simulink model "gm_Model"  (R2025a)
settings: Solver=FixedStepDiscrete  StartTime=0.0  StopTime=80000/fs_in  RelTol=1e-3
undefined symbols (not defined in the file or in its folder): a, b, b_fixp, beta_retanh, c, cos_omega, cos_omega_fixp, diag_count, exp_omega, exp_omega_fixp, fixp_chebacc_frac, fixp_chebacc_ws, fixp_dsp_ws, fixp_eig_frac, fixp_eig_ws, fs_in, group_size, hann_table_fixp, image_seed, image_seed_fixp, J_ROM, k, K_ROM, lap_diags, lap_main, lap_main_fi, lap_offsets, lap_offsets_fi, lap_rest, lap_rest_fi, laplacian_diags_main, laplacian_diags_offsets, laplacian_diags_rest, lut_norm_x, lut_norm_y, magnitude, n_ch, n_layer, n_px, n_px_fi, nf, norm_gain_floor, power_iters, power_norm_scaling_factor_fixp, tau, tau_fixp, theta, theta_fixp
libraries: simulink x59, hdlsllib x36, hdlstreaminglib x4, hdlmdlgenlib x1, matrix_library x1, dspvision x1
(part 7 of 8)

== system gm_Model/DUT_Test/Goertzel/EnabledGoertzel/crp_temp_streamed2/Serializer_Subnetwork1 ==
  in0 : Inport  OutDataTypeStr=fixdt(1, 18, 13)  PortDimensions=[1 48]  SampleTime=3.125e-07
  in1 : Inport  Port=2  OutDataTypeStr=fixdt(0, 6, 0)  SampleTime=3.125e-07
  ratechange_splitcomp : Demux  Outputs=48
  splitcomp_multiport : MultiPortSwitch  DataPortOrder=Zero-based contiguous  Inputs=48  DiagnosticForDefault=None  zeroidx=on  OutDataTypeStr=fixdt(1, 18, 13)  SampleTime=3.125e-07  SaturateOnIntegerOverflow=off  InputSameDT=off
  out0 : Outport  OutDataTypeStr=fixdt(1, 18, 13)  SampleTime=3.125e-07
  wires:
  in0/1 -> ratechange_splitcomp/1
  in1/1 -> splitcomp_multiport/1
  ratechange_splitcomp/1 -> splitcomp_multiport/2
  ratechange_splitcomp/2 -> splitcomp_multiport/3
  ratechange_splitcomp/3 -> splitcomp_multiport/4
  ratechange_splitcomp/4 -> splitcomp_multiport/5
  ratechange_splitcomp/8 -> splitcomp_multiport/9
  ratechange_splitcomp/7 -> splitcomp_multiport/8
  ratechange_splitcomp/5 -> splitcomp_multiport/6
  ratechange_splitcomp/6 -> splitcomp_multiport/7
  ratechange_splitcomp/12 -> splitcomp_multiport/13
  ratechange_splitcomp/11 -> splitcomp_multiport/12
  ratechange_splitcomp/10 -> splitcomp_multiport/11
  ratechange_splitcomp/9 -> splitcomp_multiport/10
  ratechange_splitcomp/16 -> splitcomp_multiport/17
  ratechange_splitcomp/15 -> splitcomp_multiport/16
  ratechange_splitcomp/14 -> splitcomp_multiport/15
  ratechange_splitcomp/13 -> splitcomp_multiport/14
  splitcomp_multiport/1 -> out0/1
  ratechange_splitcomp/20 -> splitcomp_multiport/21
  ratechange_splitcomp/19 -> splitcomp_multiport/20
  ratechange_splitcomp/18 -> splitcomp_multiport/19
  ratechange_splitcomp/17 -> splitcomp_multiport/18
  ratechange_splitcomp/45 -> splitcomp_multiport/46
  ratechange_splitcomp/44 -> splitcomp_multiport/45
  ratechange_splitcomp/43 -> splitcomp_multiport/44
  ratechange_splitcomp/42 -> splitcomp_multiport/43
  ratechange_splitcomp/24 -> splitcomp_multiport/25
  ratechange_splitcomp/23 -> splitcomp_multiport/24
  ratechange_splitcomp/22 -> splitcomp_multiport/23
  ratechange_splitcomp/21 -> splitcomp_multiport/22
  ratechange_splitcomp/48 -> splitcomp_multiport/49
  ratechange_splitcomp/47 -> splitcomp_multiport/48
  ratechange_splitcomp/46 -> splitcomp_multiport/47
  ratechange_splitcomp/28 -> splitcomp_multiport/29
  ratechange_splitcomp/27 -> splitcomp_multiport/28
  ratechange_splitcomp/26 -> splitcomp_multiport/27
  ratechange_splitcomp/25 -> splitcomp_multiport/26
  ratechange_splitcomp/32 -> splitcomp_multiport/33
  ratechange_splitcomp/31 -> splitcomp_multiport/32
  ratechange_splitcomp/30 -> splitcomp_multiport/31
  ratechange_splitcomp/29 -> splitcomp_multiport/30
  ratechange_splitcomp/36 -> splitcomp_multiport/37
  ratechange_splitcomp/35 -> splitcomp_multiport/36
  ratechange_splitcomp/34 -> splitcomp_multiport/35
  ratechange_splitcomp/33 -> splitcomp_multiport/34
  ratechange_splitcomp/39 -> splitcomp_multiport/40
  ratechange_splitcomp/38 -> splitcomp_multiport/39
  ratechange_splitcomp/37 -> splitcomp_multiport/38
  ratechange_splitcomp/40 -> splitcomp_multiport/41
  ratechange_splitcomp/41 -> splitcomp_multiport/42

== system gm_Model/DUT_Test/Goertzel/EnabledGoertzel/crp_temp_streamed2/Switch_out1_bypass ==
  in0 : Inport  OutDataTypeStr=fixdt(1, 18, 13)  SampleTime=3.125e-07
  in1 : Inport  Port=2  OutDataTypeStr=boolean  SampleTime=3.125e-07
  Switch_out1_enb : Switch  Criteria=u2 ~= 0  Threshold=double(0)  OutDataTypeStr=fixdt(1, 18, 13)  SampleTime=3.125e-07  SaturateOnIntegerOverflow=off  InputSameDT=off
  Switch_out1_state : Delay  DelayLength=double(1)  InitialCondition=0  SampleTime=3.125e-07
  out0 : Outport  OutDataTypeStr=fixdt(1, 18, 13)  SampleTime=3.125e-07
  wires:
  in1/1 -> Switch_out1_enb/2
  in0/1 -> Switch_out1_enb/1
  Switch_out1_state/1 -> Switch_out1_enb/3
  Switch_out1_enb/1 -> Switch_out1_state/1, out0/1

== system gm_Model/DUT_Test/Goertzel/EnabledGoertzel/crp_temp_streamed2/counter ==
  globalSchedule : EnablePort  OutDataTypeStr=boolean
  ctr_0_47 : hdlsllib/Sources/HDL Counter  CountType=Count limited  CountInit=double(0)  CountStep=double(1)  CountMax=double(47)  CountFromType=Initial value  CountFrom=double(0)  CountResetPort=off  CountLoadPort=off  CountEnbPort=off  CountDirPort=off  CountHitOutputPort=off  CountDataType=Unsigned  CountWordLen=6  CountFracLen=0  CountSampTime=3.125e-07
  out0 : Outport  OutDataTypeStr=fixdt(0, 6, 0)  SampleTime=3.125e-07  InitialOutput=0
  wires:
  ctr_0_47/1 -> out0/1

== system gm_Model/DUT_Test/Goertzel/EnabledGoertzel/crp_temp_streamed2/tappedDelay ==
  in0 : Inport  OutDataTypeStr=fixdt(1, 18, 13)  SampleTime=3.125e-07
  globalSchedule : EnablePort  OutDataTypeStr=boolean
  StateControl : StateControl  StateControl=Synchronous
  tapped_delay : simulink/Discrete/Tapped Delay  vinit=0  samptime=-1  NumDelays=double(47)  DelayOrder=Oldest  includeCurrent=off
  out0 : Outport  OutDataTypeStr=fixdt(1, 18, 13)  PortDimensions=[47]  SampleTime=3.125e-07  InitialOutput=0
  wires:
  in0/1 -> tapped_delay/1
  tapped_delay/1 -> out0/1

== system gm_Model/DUT_Test/Goertzel/EnabledGoertzel/streaming_partition_streamed/Serializer_Subnetwork ==
  in0 : Inport  OutDataTypeStr=fixdt(1, 18, 13)  PortDimensions=[1 48]  SampleTime=3.125e-07
  in1 : Inport  Port=2  OutDataTypeStr=fixdt(0, 6, 0)  SampleTime=3.125e-07
  ratechange_splitcomp : Demux  Outputs=48
  splitcomp_multiport : MultiPortSwitch  DataPortOrder=Zero-based contiguous  Inputs=48  DiagnosticForDefault=None  zeroidx=on  OutDataTypeStr=fixdt(1, 18, 13)  SampleTime=3.125e-07  SaturateOnIntegerOverflow=off  InputSameDT=off
  out0 : Outport  OutDataTypeStr=fixdt(1, 18, 13)  SampleTime=3.125e-07
  wires:
  in0/1 -> ratechange_splitcomp/1
  in1/1 -> splitcomp_multiport/1
  ratechange_splitcomp/1 -> splitcomp_multiport/2
  ratechange_splitcomp/2 -> splitcomp_multiport/3
  ratechange_splitcomp/3 -> splitcomp_multiport/4
  ratechange_splitcomp/7 -> splitcomp_multiport/8
  ratechange_splitcomp/4 -> splitcomp_multiport/5
  ratechange_splitcomp/5 -> splitcomp_multiport/6
  ratechange_splitcomp/6 -> splitcomp_multiport/7
  ratechange_splitcomp/11 -> splitcomp_multiport/12
  ratechange_splitcomp/10 -> splitcomp_multiport/11
  ratechange_splitcomp/9 -> splitcomp_multiport/10
  ratechange_splitcomp/8 -> splitcomp_multiport/9
  ratechange_splitcomp/15 -> splitcomp_multiport/16
  ratechange_splitcomp/14 -> splitcomp_multiport/15
  ratechange_splitcomp/13 -> splitcomp_multiport/14
  ratechange_splitcomp/12 -> splitcomp_multiport/13
  ratechange_splitcomp/19 -> splitcomp_multiport/20
  ratechange_splitcomp/18 -> splitcomp_multiport/19
  ratechange_splitcomp/17 -> splitcomp_multiport/18
  ratechange_splitcomp/16 -> splitcomp_multiport/17
  ratechange_splitcomp/23 -> splitcomp_multiport/24
  ratechange_splitcomp/22 -> splitcomp_multiport/23
  ratechange_splitcomp/21 -> splitcomp_multiport/22
  ratechange_splitcomp/20 -> splitcomp_multiport/21
  ratechange_splitcomp/27 -> splitcomp_multiport/28
  ratechange_splitcomp/26 -> splitcomp_multiport/27
  ratechange_splitcomp/25 -> splitcomp_multiport/26
  ratechange_splitcomp/24 -> splitcomp_multiport/25
  ratechange_splitcomp/31 -> splitcomp_multiport/32
  ratechange_splitcomp/30 -> splitcomp_multiport/31
  ratechange_splitcomp/29 -> splitcomp_multiport/30
  ratechange_splitcomp/28 -> splitcomp_multiport/29
  ratechange_splitcomp/35 -> splitcomp_multiport/36
  ratechange_splitcomp/34 -> splitcomp_multiport/35
  ratechange_splitcomp/33 -> splitcomp_multiport/34
  ratechange_splitcomp/32 -> splitcomp_multiport/33
  ratechange_splitcomp/39 -> splitcomp_multiport/40
  ratechange_splitcomp/38 -> splitcomp_multiport/39
  ratechange_splitcomp/37 -> splitcomp_multiport/38
  ratechange_splitcomp/36 -> splitcomp_multiport/37
  ratechange_splitcomp/43 -> splitcomp_multiport/44
  ratechange_splitcomp/42 -> splitcomp_multiport/43
  ratechange_splitcomp/41 -> splitcomp_multiport/42
  ratechange_splitcomp/40 -> splitcomp_multiport/41
  ratechange_splitcomp/47 -> splitcomp_multiport/48
  ratechange_splitcomp/46 -> splitcomp_multiport/47
  ratechange_splitcomp/45 -> splitcomp_multiport/46
  ratechange_splitcomp/44 -> splitcomp_multiport/45
  ratechange_splitcomp/48 -> splitcomp_multiport/49
  splitcomp_multiport/1 -> out0/1

== system gm_Model/DUT_Test/Goertzel/EnabledGoertzel/streaming_partition_streamed/Serializer_Subnetwork1 ==
  in0 : Inport  OutDataTypeStr=fixdt(1, 18, 13)  PortDimensions=[1 48]  SampleTime=3.125e-07
  in1 : Inport  Port=2  OutDataTypeStr=fixdt(0, 6, 0)  SampleTime=3.125e-07
  ratechange_splitcomp : Demux  Outputs=48
  splitcomp_multiport : MultiPortSwitch  DataPortOrder=Zero-based contiguous  Inputs=48  DiagnosticForDefault=None  zeroidx=on  OutDataTypeStr=fixdt(1, 18, 13)  SampleTime=3.125e-07  SaturateOnIntegerOverflow=off  InputSameDT=off
  out0 : Outport  OutDataTypeStr=fixdt(1, 18, 13)  SampleTime=3.125e-07
  wires:
  in0/1 -> ratechange_splitcomp/1
  in1/1 -> splitcomp_multiport/1
  ratechange_splitcomp/1 -> splitcomp_multiport/2
  ratechange_splitcomp/2 -> splitcomp_multiport/3
  ratechange_splitcomp/3 -> splitcomp_multiport/4
  ratechange_splitcomp/4 -> splitcomp_multiport/5
  ratechange_splitcomp/8 -> splitcomp_multiport/9
  ratechange_splitcomp/7 -> splitcomp_multiport/8
  ratechange_splitcomp/5 -> splitcomp_multiport/6
  ratechange_splitcomp/6 -> splitcomp_multiport/7
  ratechange_splitcomp/12 -> splitcomp_multiport/13
  ratechange_splitcomp/11 -> splitcomp_multiport/12
  ratechange_splitcomp/10 -> splitcomp_multiport/11
  ratechange_splitcomp/9 -> splitcomp_multiport/10
  ratechange_splitcomp/16 -> splitcomp_multiport/17
  ratechange_splitcomp/15 -> splitcomp_multiport/16
  ratechange_splitcomp/14 -> splitcomp_multiport/15
  ratechange_splitcomp/13 -> splitcomp_multiport/14
  ratechange_splitcomp/20 -> splitcomp_multiport/21
  ratechange_splitcomp/19 -> splitcomp_multiport/20
  ratechange_splitcomp/18 -> splitcomp_multiport/19
  ratechange_splitcomp/17 -> splitcomp_multiport/18
  ratechange_splitcomp/24 -> splitcomp_multiport/25
  ratechange_splitcomp/23 -> splitcomp_multiport/24
  ratechange_splitcomp/22 -> splitcomp_multiport/23
  ratechange_splitcomp/21 -> splitcomp_multiport/22
  ratechange_splitcomp/28 -> splitcomp_multiport/29
  ratechange_splitcomp/27 -> splitcomp_multiport/28
  ratechange_splitcomp/26 -> splitcomp_multiport/27
  ratechange_splitcomp/25 -> splitcomp_multiport/26
  ratechange_splitcomp/32 -> splitcomp_multiport/33
  ratechange_splitcomp/31 -> splitcomp_multiport/32
  ratechange_splitcomp/30 -> splitcomp_multiport/31
  ratechange_splitcomp/29 -> splitcomp_multiport/30
  ratechange_splitcomp/36 -> splitcomp_multiport/37
  ratechange_splitcomp/35 -> splitcomp_multiport/36
  ratechange_splitcomp/34 -> splitcomp_multiport/35
  ratechange_splitcomp/33 -> splitcomp_multiport/34
  ratechange_splitcomp/39 -> splitcomp_multiport/40
  ratechange_splitcomp/38 -> splitcomp_multiport/39
  ratechange_splitcomp/37 -> splitcomp_multiport/38
  ratechange_splitcomp/40 -> splitcomp_multiport/41
  ratechange_splitcomp/41 -> splitcomp_multiport/42
  ratechange_splitcomp/45 -> splitcomp_multiport/46
  ratechange_splitcomp/44 -> splitcomp_multiport/45
  ratechange_splitcomp/43 -> splitcomp_multiport/44
  ratechange_splitcomp/42 -> splitcomp_multiport/43
  ratechange_splitcomp/48 -> splitcomp_multiport/49
  ratechange_splitcomp/47 -> splitcomp_multiport/48
  ratechange_splitcomp/46 -> splitcomp_multiport/47
  splitcomp_multiport/1 -> out0/1

== system gm_Model/DUT_Test/Goertzel/EnabledGoertzel/streaming_partition_streamed/Serializer_Subnetwork2 ==
  in0 : Inport  OutDataTypeStr=fixdt(1, 12, 11)  PortDimensions=[1 48]  SampleTime=3.125e-07
  in1 : Inport  Port=2  OutDataTypeStr=fixdt(0, 6, 0)  SampleTime=3.125e-07
  ratechange_splitcomp : Demux  Outputs=48
  splitcomp_multiport : MultiPortSwitch  DataPortOrder=Zero-based contiguous  Inputs=48  DiagnosticForDefault=None  zeroidx=on  OutDataTypeStr=fixdt(1, 12, 11)  SampleTime=3.125e-07  SaturateOnIntegerOverflow=off  InputSameDT=off
  out0 : Outport  OutDataTypeStr=fixdt(1, 12, 11)  SampleTime=3.125e-07
  wires:
  ratechange_splitcomp/47 -> splitcomp_multiport/48
  ratechange_splitcomp/46 -> splitcomp_multiport/47
  ratechange_splitcomp/45 -> splitcomp_multiport/46
  ratechange_splitcomp/44 -> splitcomp_multiport/45
  in0/1 -> ratechange_splitcomp/1
  in1/1 -> splitcomp_multiport/1
  ratechange_splitcomp/1 -> splitcomp_multiport/2
  ratechange_splitcomp/2 -> splitcomp_multiport/3
  ratechange_splitcomp/43 -> splitcomp_multiport/44
  ratechange_splitcomp/42 -> splitcomp_multiport/43
  ratechange_splitcomp/3 -> splitcomp_multiport/4
  ratechange_splitcomp/4 -> splitcomp_multiport/5
  ratechange_splitcomp/5 -> splitcomp_multiport/6
  ratechange_splitcomp/6 -> splitcomp_multiport/7
  ratechange_splitcomp/10 -> splitcomp_multiport/11
  ratechange_splitcomp/9 -> splitcomp_multiport/10
  ratechange_splitcomp/8 -> splitcomp_multiport/9
  ratechange_splitcomp/7 -> splitcomp_multiport/8
  ratechange_splitcomp/14 -> splitcomp_multiport/15
  ratechange_splitcomp/13 -> splitcomp_multiport/14
  ratechange_splitcomp/12 -> splitcomp_multiport/13
  ratechange_splitcomp/11 -> splitcomp_multiport/12
  splitcomp_multiport/1 -> out0/1
  ratechange_splitcomp/18 -> splitcomp_multiport/19
  ratechange_splitcomp/17 -> splitcomp_multiport/18
  ratechange_splitcomp/16 -> splitcomp_multiport/17
  ratechange_splitcomp/15 -> splitcomp_multiport/16
  ratechange_splitcomp/22 -> splitcomp_multiport/23
  ratechange_splitcomp/21 -> splitcomp_multiport/22
  ratechange_splitcomp/20 -> splitcomp_multiport/21
  ratechange_splitcomp/19 -> splitcomp_multiport/20
  ratechange_splitcomp/26 -> splitcomp_multiport/27
  ratechange_splitcomp/25 -> splitcomp_multiport/26
  ratechange_splitcomp/24 -> splitcomp_multiport/25
  ratechange_splitcomp/23 -> splitcomp_multiport/24
  ratechange_splitcomp/30 -> splitcomp_multiport/31
  ratechange_splitcomp/29 -> splitcomp_multiport/30
  ratechange_splitcomp/28 -> splitcomp_multiport/29
  ratechange_splitcomp/27 -> splitcomp_multiport/28
  ratechange_splitcomp/34 -> splitcomp_multiport/35
  ratechange_splitcomp/33 -> splitcomp_multiport/34
  ratechange_splitcomp/32 -> splitcomp_multiport/33
  ratechange_splitcomp/31 -> splitcomp_multiport/32
  ratechange_splitcomp/38 -> splitcomp_multiport/39
  ratechange_splitcomp/37 -> splitcomp_multiport/38
  ratechange_splitcomp/36 -> splitcomp_multiport/37
  ratechange_splitcomp/35 -> splitcomp_multiport/36
  ratechange_splitcomp/39 -> splitcomp_multiport/40
  ratechange_splitcomp/40 -> splitcomp_multiport/41
  ratechange_splitcomp/41 -> splitcomp_multiport/42
  ratechange_splitcomp/48 -> splitcomp_multiport/49

== system gm_Model/DUT_Test/Goertzel/EnabledGoertzel/streaming_partition_streamed/Serializer_Subnetwork3 ==
  in0 : Inport  OutDataTypeStr=fixdt(1, 18, 13)  PortDimensions=[1 48]  SampleTime=3.125e-07
  in1 : Inport  Port=2  OutDataTypeStr=fixdt(0, 6, 0)  SampleTime=3.125e-07
  ratechange_splitcomp : Demux  Outputs=48
  splitcomp_multiport : MultiPortSwitch  DataPortOrder=Zero-based contiguous  Inputs=48  DiagnosticForDefault=None  zeroidx=on  OutDataTypeStr=fixdt(1, 18, 13)  SampleTime=3.125e-07  SaturateOnIntegerOverflow=off  InputSameDT=off
  out0 : Outport  OutDataTypeStr=fixdt(1, 18, 13)  SampleTime=3.125e-07
  wires:
  in0/1 -> ratechange_splitcomp/1
  in1/1 -> splitcomp_multiport/1
  ratechange_splitcomp/1 -> splitcomp_multiport/2
  ratechange_splitcomp/2 -> splitcomp_multiport/3
  ratechange_splitcomp/3 -> splitcomp_multiport/4
  ratechange_splitcomp/4 -> splitcomp_multiport/5
  ratechange_splitcomp/8 -> splitcomp_multiport/9
  ratechange_splitcomp/7 -> splitcomp_multiport/8
  ratechange_splitcomp/5 -> splitcomp_multiport/6
  ratechange_splitcomp/6 -> splitcomp_multiport/7
  ratechange_splitcomp/12 -> splitcomp_multiport/13
  ratechange_splitcomp/11 -> splitcomp_multiport/12
  ratechange_splitcomp/10 -> splitcomp_multiport/11
  ratechange_splitcomp/9 -> splitcomp_multiport/10
  ratechange_splitcomp/16 -> splitcomp_multiport/17
  ratechange_splitcomp/15 -> splitcomp_multiport/16
  ratechange_splitcomp/14 -> splitcomp_multiport/15
  ratechange_splitcomp/13 -> splitcomp_multiport/14
  ratechange_splitcomp/20 -> splitcomp_multiport/21
  ratechange_splitcomp/19 -> splitcomp_multiport/20
  ratechange_splitcomp/18 -> splitcomp_multiport/19
  ratechange_splitcomp/17 -> splitcomp_multiport/18
  ratechange_splitcomp/24 -> splitcomp_multiport/25
  ratechange_splitcomp/23 -> splitcomp_multiport/24
  ratechange_splitcomp/22 -> splitcomp_multiport/23
  ratechange_splitcomp/21 -> splitcomp_multiport/22
  ratechange_splitcomp/28 -> splitcomp_multiport/29
  ratechange_splitcomp/27 -> splitcomp_multiport/28
  ratechange_splitcomp/26 -> splitcomp_multiport/27
  ratechange_splitcomp/25 -> splitcomp_multiport/26
  ratechange_splitcomp/32 -> splitcomp_multiport/33
  ratechange_splitcomp/31 -> splitcomp_multiport/32
  ratechange_splitcomp/30 -> splitcomp_multiport/31
  ratechange_splitcomp/29 -> splitcomp_multiport/30
  ratechange_splitcomp/36 -> splitcomp_multiport/37
  ratechange_splitcomp/35 -> splitcomp_multiport/36
  ratechange_splitcomp/34 -> splitcomp_multiport/35
  ratechange_splitcomp/33 -> splitcomp_multiport/34
  ratechange_splitcomp/39 -> splitcomp_multiport/40
  ratechange_splitcomp/38 -> splitcomp_multiport/39
  ratechange_splitcomp/37 -> splitcomp_multiport/38
  ratechange_splitcomp/40 -> splitcomp_multiport/41
  ratechange_splitcomp/41 -> splitcomp_multiport/42
  ratechange_splitcomp/45 -> splitcomp_multiport/46
  ratechange_splitcomp/44 -> splitcomp_multiport/45
  ratechange_splitcomp/43 -> splitcomp_multiport/44
  ratechange_splitcomp/42 -> splitcomp_multiport/43
  ratechange_splitcomp/48 -> splitcomp_multiport/49
  ratechange_splitcomp/47 -> splitcomp_multiport/48
  ratechange_splitcomp/46 -> splitcomp_multiport/47
  splitcomp_multiport/1 -> out0/1

== system gm_Model/DUT_Test/Goertzel/EnabledGoertzel/streaming_partition_streamed/Serializer_Subnetwork4 ==
  in0 : Inport  OutDataTypeStr=fixdt(1, 18, 13)  PortDimensions=[1 48]  SampleTime=3.125e-07
  in1 : Inport  Port=2  OutDataTypeStr=fixdt(0, 6, 0)  SampleTime=3.125e-07
  ratechange_splitcomp : Demux  Outputs=48
  splitcomp_multiport : MultiPortSwitch  DataPortOrder=Zero-based contiguous  Inputs=48  DiagnosticForDefault=None  zeroidx=on  OutDataTypeStr=fixdt(1, 18, 13)  SampleTime=3.125e-07  SaturateOnIntegerOverflow=off  InputSameDT=off
  out0 : Outport  OutDataTypeStr=fixdt(1, 18, 13)  SampleTime=3.125e-07
  wires:
  ratechange_splitcomp/47 -> splitcomp_multiport/48
  ratechange_splitcomp/46 -> splitcomp_multiport/47
  ratechange_splitcomp/45 -> splitcomp_multiport/46
  ratechange_splitcomp/44 -> splitcomp_multiport/45
  in0/1 -> ratechange_splitcomp/1
  in1/1 -> splitcomp_multiport/1
  ratechange_splitcomp/1 -> splitcomp_multiport/2
  ratechange_splitcomp/2 -> splitcomp_multiport/3
  ratechange_splitcomp/3 -> splitcomp_multiport/4
  ratechange_splitcomp/4 -> splitcomp_multiport/5
  ratechange_splitcomp/5 -> splitcomp_multiport/6
  ratechange_splitcomp/6 -> splitcomp_multiport/7
  ratechange_splitcomp/10 -> splitcomp_multiport/11
  ratechange_splitcomp/9 -> splitcomp_multiport/10
  ratechange_splitcomp/8 -> splitcomp_multiport/9
  ratechange_splitcomp/7 -> splitcomp_multiport/8
  ratechange_splitcomp/48 -> splitcomp_multiport/49
  ratechange_splitcomp/14 -> splitcomp_multiport/15
  ratechange_splitcomp/13 -> splitcomp_multiport/14
  ratechange_splitcomp/12 -> splitcomp_multiport/13
  ratechange_splitcomp/11 -> splitcomp_multiport/12
  splitcomp_multiport/1 -> out0/1
  ratechange_splitcomp/18 -> splitcomp_multiport/19
  ratechange_splitcomp/17 -> splitcomp_multiport/18
  ratechange_splitcomp/16 -> splitcomp_multiport/17
  ratechange_splitcomp/15 -> splitcomp_multiport/16
  ratechange_splitcomp/22 -> splitcomp_multiport/23
  ratechange_splitcomp/21 -> splitcomp_multiport/22
  ratechange_splitcomp/20 -> splitcomp_multiport/21
  ratechange_splitcomp/19 -> splitcomp_multiport/20
  ratechange_splitcomp/26 -> splitcomp_multiport/27
  ratechange_splitcomp/25 -> splitcomp_multiport/26
  ratechange_splitcomp/24 -> splitcomp_multiport/25
  ratechange_splitcomp/23 -> splitcomp_multiport/24
  ratechange_splitcomp/30 -> splitcomp_multiport/31
  ratechange_splitcomp/29 -> splitcomp_multiport/30
  ratechange_splitcomp/28 -> splitcomp_multiport/29
  ratechange_splitcomp/27 -> splitcomp_multiport/28
  ratechange_splitcomp/34 -> splitcomp_multiport/35
  ratechange_splitcomp/33 -> splitcomp_multiport/34
  ratechange_splitcomp/32 -> splitcomp_multiport/33
  ratechange_splitcomp/31 -> splitcomp_multiport/32
  ratechange_splitcomp/40 -> splitcomp_multiport/41
  ratechange_splitcomp/38 -> splitcomp_multiport/39
  ratechange_splitcomp/37 -> splitcomp_multiport/38
  ratechange_splitcomp/36 -> splitcomp_multiport/37
  ratechange_splitcomp/35 -> splitcomp_multiport/36
  ratechange_splitcomp/39 -> splitcomp_multiport/40
  ratechange_splitcomp/41 -> splitcomp_multiport/42
  ratechange_splitcomp/43 -> splitcomp_multiport/44
  ratechange_splitcomp/42 -> splitcomp_multiport/43

== system gm_Model/DUT_Test/Goertzel/EnabledGoertzel/streaming_partition_streamed/Switch1_out1_bypass ==
  in0 : Inport  OutDataTypeStr=fixdt(1, 18, 13)  SampleTime=3.125e-07
  in1 : Inport  Port=2  OutDataTypeStr=boolean  SampleTime=3.125e-07
  Switch1_out1_enb : Switch  Criteria=u2 ~= 0  Threshold=double(0)  OutDataTypeStr=fixdt(1, 18, 13)  SampleTime=3.125e-07  SaturateOnIntegerOverflow=off  InputSameDT=off
  Switch1_out1_state : Delay  DelayLength=double(1)  InitialCondition=0  SampleTime=3.125e-07
  out0 : Outport  OutDataTypeStr=fixdt(1, 18, 13)  SampleTime=3.125e-07
  wires:
  in0/1 -> Switch1_out1_enb/1
  in1/1 -> Switch1_out1_enb/2
  Switch1_out1_state/1 -> Switch1_out1_enb/3
  Switch1_out1_enb/1 -> Switch1_out1_state/1, out0/1

== system gm_Model/DUT_Test/Goertzel/EnabledGoertzel/streaming_partition_streamed/Switch1_out1_bypass1 ==
  in0 : Inport  OutDataTypeStr=fixdt(1, 18, 13)  SampleTime=3.125e-07
  in1 : Inport  Port=2  OutDataTypeStr=boolean  SampleTime=3.125e-07
  Switch1_out1_enb : Switch  Criteria=u2 ~= 0  Threshold=double(0)  OutDataTypeStr=fixdt(1, 18, 13)  SampleTime=3.125e-07  SaturateOnIntegerOverflow=off  InputSameDT=off
  Switch1_out1_state : Delay  DelayLength=double(1)  InitialCondition=0  SampleTime=3.125e-07
  out0 : Outport  OutDataTypeStr=fixdt(1, 18, 13)  SampleTime=3.125e-07
  wires:
  in0/1 -> Switch1_out1_enb/1
  in1/1 -> Switch1_out1_enb/2
  Switch1_out1_state/1 -> Switch1_out1_enb/3
  Switch1_out1_enb/1 -> Switch1_out1_state/1, out0/1

== system gm_Model/DUT_Test/Goertzel/EnabledGoertzel/streaming_partition_streamed/counter ==
  globalSchedule : EnablePort  OutDataTypeStr=boolean
  ctr_0_47 : hdlsllib/Sources/HDL Counter  CountType=Count limited  CountInit=double(0)  CountStep=double(1)  CountMax=double(47)  CountFromType=Initial value  CountFrom=double(0)  CountResetPort=off  CountLoadPort=off  CountEnbPort=off  CountDirPort=off  CountHitOutputPort=off  CountDataType=Unsigned  CountWordLen=6  CountFracLen=0  CountSampTime=3.125e-07
  out0 : Outport  OutDataTypeStr=fixdt(0, 6, 0)  SampleTime=3.125e-07  InitialOutput=0
  wires:
  ctr_0_47/1 -> out0/1

== system gm_Model/DUT_Test/Goertzel/EnabledGoertzel/streaming_partition_streamed/tappedDelay ==
  in0 : Inport  OutDataTypeStr=fixdt(1, 18, 13)  SampleTime=3.125e-07
  globalSchedule : EnablePort  OutDataTypeStr=boolean
  StateControl : StateControl  StateControl=Synchronous
  tapped_delay : simulink/Discrete/Tapped Delay  vinit=0  samptime=-1  NumDelays=double(47)  DelayOrder=Oldest  includeCurrent=off
  out0 : Outport  OutDataTypeStr=fixdt(1, 18, 13)  PortDimensions=[47]  SampleTime=3.125e-07  InitialOutput=0
  wires:
  in0/1 -> tapped_delay/1
  tapped_delay/1 -> out0/1

== system gm_Model/DUT_Test/Goertzel/EnabledGoertzel/streaming_partition_streamed/tappedDelay1 ==
  in0 : Inport  OutDataTypeStr=fixdt(1, 18, 13)  SampleTime=3.125e-07
  globalSchedule : EnablePort  OutDataTypeStr=boolean
  StateControl : StateControl  StateControl=Synchronous
  tapped_delay : simulink/Discrete/Tapped Delay  vinit=0  samptime=-1  NumDelays=double(47)  DelayOrder=Oldest  includeCurrent=off
  out0 : Outport  OutDataTypeStr=fixdt(1, 18, 13)  PortDimensions=[47]  SampleTime=3.125e-07  InitialOutput=0
  wires:
  in0/1 -> tapped_delay/1
  tapped_delay/1 -> out0/1

== system gm_Model/DUT_Test/Goertzel/EnabledGoertzel/streaming_partition_streamed1/Serializer_Subnetwork ==
  in0 : Inport  OutDataTypeStr=fixdt(1, 18, 13)  PortDimensions=[1 48]  SampleTime=3.125e-07
      settings: SignalType=complex
  in1 : Inport  Port=2  OutDataTypeStr=fixdt(0, 6, 0)  SampleTime=3.125e-07
  ratechange_splitcomp : Demux  Outputs=48
  splitcomp_multiport : MultiPortSwitch  DataPortOrder=Zero-based contiguous  Inputs=48  DiagnosticForDefault=None  zeroidx=on  OutDataTypeStr=fixdt(1, 18, 13)  SampleTime=3.125e-07  SaturateOnIntegerOverflow=off  InputSameDT=off
  out0 : Outport  OutDataTypeStr=fixdt(1, 18, 13)  SampleTime=3.125e-07
      settings: SignalType=complex
  wires:
  in0/1 -> ratechange_splitcomp/1
  in1/1 -> splitcomp_multiport/1
  ratechange_splitcomp/1 -> splitcomp_multiport/2
  ratechange_splitcomp/3 -> splitcomp_multiport/4
  ratechange_splitcomp/5 -> splitcomp_multiport/6
  ratechange_splitcomp/2 -> splitcomp_multiport/3
  ratechange_splitcomp/4 -> splitcomp_multiport/5
  ratechange_splitcomp/12 -> splitcomp_multiport/13
  ratechange_splitcomp/10 -> splitcomp_multiport/11
  ratechange_splitcomp/8 -> splitcomp_multiport/9
  ratechange_splitcomp/6 -> splitcomp_multiport/7
  ratechange_splitcomp/13 -> splitcomp_multiport/14
  ratechange_splitcomp/11 -> splitcomp_multiport/12
  ratechange_splitcomp/9 -> splitcomp_multiport/10
  ratechange_splitcomp/7 -> splitcomp_multiport/8
  ratechange_splitcomp/20 -> splitcomp_multiport/21
  ratechange_splitcomp/18 -> splitcomp_multiport/19
  ratechange_splitcomp/16 -> splitcomp_multiport/17
  ratechange_splitcomp/14 -> splitcomp_multiport/15
  ratechange_splitcomp/21 -> splitcomp_multiport/22
  ratechange_splitcomp/19 -> splitcomp_multiport/20
  ratechange_splitcomp/17 -> splitcomp_multiport/18
  ratechange_splitcomp/15 -> splitcomp_multiport/16
  ratechange_splitcomp/28 -> splitcomp_multiport/29
  ratechange_splitcomp/26 -> splitcomp_multiport/27
  ratechange_splitcomp/24 -> splitcomp_multiport/25
  ratechange_splitcomp/22 -> splitcomp_multiport/23
  ratechange_splitcomp/29 -> splitcomp_multiport/30
  ratechange_splitcomp/27 -> splitcomp_multiport/28
  ratechange_splitcomp/25 -> splitcomp_multiport/26
  ratechange_splitcomp/23 -> splitcomp_multiport/24
  ratechange_splitcomp/36 -> splitcomp_multiport/37
  ratechange_splitcomp/34 -> splitcomp_multiport/35
  ratechange_splitcomp/32 -> splitcomp_multiport/33
  ratechange_splitcomp/30 -> splitcomp_multiport/31
  ratechange_splitcomp/37 -> splitcomp_multiport/38
  ratechange_splitcomp/35 -> splitcomp_multiport/36
  ratechange_splitcomp/33 -> splitcomp_multiport/34
  ratechange_splitcomp/31 -> splitcomp_multiport/32
  ratechange_splitcomp/44 -> splitcomp_multiport/45
  ratechange_splitcomp/42 -> splitcomp_multiport/43
  ratechange_splitcomp/40 -> splitcomp_multiport/41
  ratechange_splitcomp/38 -> splitcomp_multiport/39
  ratechange_splitcomp/45 -> splitcomp_multiport/46
  ratechange_splitcomp/43 -> splitcomp_multiport/44
  ratechange_splitcomp/41 -> splitcomp_multiport/42
  ratechange_splitcomp/39 -> splitcomp_multiport/40
  ratechange_splitcomp/48 -> splitcomp_multiport/49
  ratechange_splitcomp/46 -> splitcomp_multiport/47
  ratechange_splitcomp/47 -> splitcomp_multiport/48
  splitcomp_multiport/1 -> out0/1

== system gm_Model/DUT_Test/Goertzel/EnabledGoertzel/streaming_partition_streamed1/Serializer_Subnetwork1 ==
  in0 : Inport  OutDataTypeStr=fixdt(1, 18, 13)  PortDimensions=[1 48]  SampleTime=3.125e-07
      settings: SignalType=complex
  in1 : Inport  Port=2  OutDataTypeStr=fixdt(0, 6, 0)  SampleTime=3.125e-07
  ratechange_splitcomp : Demux  Outputs=48
  splitcomp_multiport : MultiPortSwitch  DataPortOrder=Zero-based contiguous  Inputs=48  DiagnosticForDefault=None  zeroidx=on  OutDataTypeStr=fixdt(1, 18, 13)  SampleTime=3.125e-07  SaturateOnIntegerOverflow=off  InputSameDT=off
  out0 : Outport  OutDataTypeStr=fixdt(1, 18, 13)  SampleTime=3.125e-07
      settings: SignalType=complex
  wires:
  in1/1 -> splitcomp_multiport/1
  in0/1 -> ratechange_splitcomp/1
  ratechange_splitcomp/2 -> splitcomp_multiport/3
  ratechange_splitcomp/4 -> splitcomp_multiport/5
  ratechange_splitcomp/6 -> splitcomp_multiport/7
  ratechange_splitcomp/1 -> splitcomp_multiport/2
  ratechange_splitcomp/3 -> splitcomp_multiport/4
  ratechange_splitcomp/5 -> splitcomp_multiport/6
  ratechange_splitcomp/13 -> splitcomp_multiport/14
  ratechange_splitcomp/11 -> splitcomp_multiport/12
  ratechange_splitcomp/9 -> splitcomp_multiport/10
  ratechange_splitcomp/7 -> splitcomp_multiport/8
  ratechange_splitcomp/41 -> splitcomp_multiport/42
  ratechange_splitcomp/14 -> splitcomp_multiport/15
  ratechange_splitcomp/12 -> splitcomp_multiport/13
  ratechange_splitcomp/10 -> splitcomp_multiport/11
  ratechange_splitcomp/8 -> splitcomp_multiport/9
  ratechange_splitcomp/21 -> splitcomp_multiport/22
  ratechange_splitcomp/19 -> splitcomp_multiport/20
  ratechange_splitcomp/17 -> splitcomp_multiport/18
  ratechange_splitcomp/15 -> splitcomp_multiport/16
  ratechange_splitcomp/22 -> splitcomp_multiport/23
  ratechange_splitcomp/20 -> splitcomp_multiport/21
  ratechange_splitcomp/18 -> splitcomp_multiport/19
  ratechange_splitcomp/16 -> splitcomp_multiport/17
  ratechange_splitcomp/29 -> splitcomp_multiport/30
  ratechange_splitcomp/27 -> splitcomp_multiport/28
  ratechange_splitcomp/25 -> splitcomp_multiport/26
  ratechange_splitcomp/23 -> splitcomp_multiport/24
  ratechange_splitcomp/30 -> splitcomp_multiport/31
  ratechange_splitcomp/28 -> splitcomp_multiport/29
  ratechange_splitcomp/26 -> splitcomp_multiport/27
  ratechange_splitcomp/24 -> splitcomp_multiport/25
  ratechange_splitcomp/37 -> splitcomp_multiport/38
  ratechange_splitcomp/35 -> splitcomp_multiport/36
  ratechange_splitcomp/33 -> splitcomp_multiport/34
  ratechange_splitcomp/31 -> splitcomp_multiport/32
  ratechange_splitcomp/38 -> splitcomp_multiport/39
  ratechange_splitcomp/36 -> splitcomp_multiport/37
  ratechange_splitcomp/34 -> splitcomp_multiport/35
  ratechange_splitcomp/32 -> splitcomp_multiport/33
  ratechange_splitcomp/39 -> splitcomp_multiport/40
  ratechange_splitcomp/40 -> splitcomp_multiport/41
  ratechange_splitcomp/42 -> splitcomp_multiport/43
  ratechange_splitcomp/43 -> splitcomp_multiport/44
  ratechange_splitcomp/48 -> splitcomp_multiport/49
  ratechange_splitcomp/46 -> splitcomp_multiport/47
  ratechange_splitcomp/44 -> splitcomp_multiport/45
  ratechange_splitcomp/47 -> splitcomp_multiport/48
  ratechange_splitcomp/45 -> splitcomp_multiport/46
  splitcomp_multiport/1 -> out0/1

== system gm_Model/DUT_Test/Goertzel/EnabledGoertzel/streaming_partition_streamed1/Sum of Elements_out1_bypass ==
  in0 : Inport  OutDataTypeStr=fixdt(1, 18, 13)  SampleTime=3.125e-07
      settings: SignalType=complex
  in1 : Inport  Port=2  OutDataTypeStr=boolean  SampleTime=3.125e-07
  Sum of Elements_out1_enb : Switch  Criteria=u2 ~= 0  Threshold=double(0)  OutDataTypeStr=fixdt(1, 18, 13)  SampleTime=3.125e-07  SaturateOnIntegerOverflow=off  InputSameDT=off
  Sum of Elements_out1_state : Delay  DelayLength=double(1)  InitialCondition=0  SampleTime=3.125e-07
  out0 : Outport  OutDataTypeStr=fixdt(1, 18, 13)  SampleTime=3.125e-07
      settings: SignalType=complex
  wires:
  in1/1 -> Sum of Elements_out1_enb/2
  in0/1 -> Sum of Elements_out1_enb/1
  Sum of Elements_out1_state/1 -> Sum of Elements_out1_enb/3
  Sum of Elements_out1_enb/1 -> out0/1, Sum of Elements_out1_state/1

== system gm_Model/DUT_Test/Goertzel/EnabledGoertzel/streaming_partition_streamed1/counter ==
  globalSchedule : EnablePort  OutDataTypeStr=boolean
  ctr_0_47 : hdlsllib/Sources/HDL Counter  CountType=Count limited  CountInit=double(0)  CountStep=double(1)  CountMax=double(47)  CountFromType=Initial value  CountFrom=double(0)  CountResetPort=off  CountLoadPort=off  CountEnbPort=off  CountDirPort=off  CountHitOutputPort=off  CountDataType=Unsigned  CountWordLen=6  CountFracLen=0  CountSampTime=3.125e-07
  out0 : Outport  OutDataTypeStr=fixdt(0, 6, 0)  SampleTime=3.125e-07  InitialOutput=0
  wires:
  ctr_0_47/1 -> out0/1

== system gm_Model/DUT_Test/Goertzel/EnabledGoertzel/streaming_partition_streamed1/tappedDelay ==
  in0 : Inport  OutDataTypeStr=fixdt(1, 18, 13)  SampleTime=3.125e-07
      settings: SignalType=complex
  globalSchedule : EnablePort  OutDataTypeStr=boolean
  StateControl : StateControl  StateControl=Synchronous
  tapped_delay : simulink/Discrete/Tapped Delay  vinit=0  samptime=-1  NumDelays=double(47)  DelayOrder=Oldest  includeCurrent=off
  out0 : Outport  OutDataTypeStr=fixdt(1, 18, 13)  PortDimensions=[47]  SampleTime=3.125e-07  InitialOutput=0
      settings: SignalType=complex
  wires:
  in0/1 -> tapped_delay/1
  tapped_delay/1 -> out0/1

== system gm_Model/DUT_Test/Goertzel/EnabledGoertzel/streaming_partition_streamed2/Multiply-Add_out1_0_bypass ==
  in0 : Inport  OutDataTypeStr=fixdt(1, 18, 13)  SampleTime=3.125e-07
      settings: SignalType=complex
  in1 : Inport  Port=2  OutDataTypeStr=boolean  SampleTime=3.125e-07
  Multiply-Add_out1_0_enb : Switch  Criteria=u2 ~= 0  Threshold=double(0)  OutDataTypeStr=fixdt(1, 18, 13)  SampleTime=3.125e-07  SaturateOnIntegerOverflow=off  InputSameDT=off
  Multiply-Add_out1_0_state : Delay  DelayLength=double(1)  InitialCondition=0  SampleTime=3.125e-07
  out0 : Outport  OutDataTypeStr=fixdt(1, 18, 13)  SampleTime=3.125e-07
      settings: SignalType=complex
  wires:
  in0/1 -> Multiply-Add_out1_0_enb/1
  in1/1 -> Multiply-Add_out1_0_enb/2
  Multiply-Add_out1_0_state/1 -> Multiply-Add_out1_0_enb/3
  Multiply-Add_out1_0_enb/1 -> Multiply-Add_out1_0_state/1, out0/1

== system gm_Model/DUT_Test/Goertzel/EnabledGoertzel/streaming_partition_streamed2/Multiply-Add_out1_1_bypass ==
  in0 : Inport  OutDataTypeStr=fixdt(1, 18, 13)  SampleTime=3.125e-07
      settings: SignalType=complex
  in1 : Inport  Port=2  OutDataTypeStr=boolean  SampleTime=3.125e-07
  Multiply-Add_out1_1_enb : Switch  Criteria=u2 ~= 0  Threshold=double(0)  OutDataTypeStr=fixdt(1, 18, 13)  SampleTime=3.125e-07  SaturateOnIntegerOverflow=off  InputSameDT=off
  Multiply-Add_out1_1_state : Delay  DelayLength=double(1)  InitialCondition=0  SampleTime=3.125e-07
  out0 : Outport  OutDataTypeStr=fixdt(1, 18, 13)  SampleTime=3.125e-07
      settings: SignalType=complex
  wires:
  in1/1 -> Multiply-Add_out1_1_enb/2
  in0/1 -> Multiply-Add_out1_1_enb/1
  Multiply-Add_out1_1_state/1 -> Multiply-Add_out1_1_enb/3
  Multiply-Add_out1_1_enb/1 -> Multiply-Add_out1_1_state/1, out0/1

== system gm_Model/DUT_Test/Goertzel/EnabledGoertzel/streaming_partition_streamed2/Serializer_Subnetwork ==
  in0 : Inport  OutDataTypeStr=fixdt(1, 18, 13)  PortDimensions=[1 48]  SampleTime=3.125e-07
  in1 : Inport  Port=2  OutDataTypeStr=fixdt(0, 6, 0)  SampleTime=3.125e-07
  ratechange_splitcomp : Demux  Outputs=48
  splitcomp_multiport : MultiPortSwitch  DataPortOrder=Zero-based contiguous  Inputs=48  DiagnosticForDefault=None  zeroidx=on  OutDataTypeStr=fixdt(1, 18, 13)  SampleTime=3.125e-07  SaturateOnIntegerOverflow=off  InputSameDT=off
  out0 : Outport  OutDataTypeStr=fixdt(1, 18, 13)  SampleTime=3.125e-07
  wires:
  ratechange_splitcomp/31 -> splitcomp_multiport/32
  ratechange_splitcomp/29 -> splitcomp_multiport/30
  ratechange_splitcomp/27 -> splitcomp_multiport/28
  ratechange_splitcomp/25 -> splitcomp_multiport/26
  in0/1 -> ratechange_splitcomp/1
  in1/1 -> splitcomp_multiport/1
  ratechange_splitcomp/2 -> splitcomp_multiport/3
  ratechange_splitcomp/4 -> splitcomp_multiport/5
  ratechange_splitcomp/6 -> splitcomp_multiport/7
  ratechange_splitcomp/7 -> splitcomp_multiport/8
  ratechange_splitcomp/1 -> splitcomp_multiport/2
  ratechange_splitcomp/3 -> splitcomp_multiport/4
  ratechange_splitcomp/5 -> splitcomp_multiport/6
  ratechange_splitcomp/14 -> splitcomp_multiport/15
  ratechange_splitcomp/12 -> splitcomp_multiport/13
  ratechange_splitcomp/10 -> splitcomp_multiport/11
  ratechange_splitcomp/8 -> splitcomp_multiport/9
  ratechange_splitcomp/15 -> splitcomp_multiport/16
  ratechange_splitcomp/13 -> splitcomp_multiport/14
  ratechange_splitcomp/11 -> splitcomp_multiport/12
  ratechange_splitcomp/9 -> splitcomp_multiport/10
  ratechange_splitcomp/22 -> splitcomp_multiport/23
  ratechange_splitcomp/20 -> splitcomp_multiport/21
  ratechange_splitcomp/18 -> splitcomp_multiport/19
  ratechange_splitcomp/16 -> splitcomp_multiport/17
  ratechange_splitcomp/23 -> splitcomp_multiport/24
  ratechange_splitcomp/21 -> splitcomp_multiport/22
  ratechange_splitcomp/19 -> splitcomp_multiport/20
  ratechange_splitcomp/17 -> splitcomp_multiport/18
  ratechange_splitcomp/30 -> splitcomp_multiport/31
  ratechange_splitcomp/28 -> splitcomp_multiport/29
  ratechange_splitcomp/26 -> splitcomp_multiport/27
  ratechange_splitcomp/24 -> splitcomp_multiport/25
  ratechange_splitcomp/38 -> splitcomp_multiport/39
  ratechange_splitcomp/36 -> splitcomp_multiport/37
  ratechange_splitcomp/34 -> splitcomp_multiport/35
  ratechange_splitcomp/32 -> splitcomp_multiport/33
  ratechange_splitcomp/39 -> splitcomp_multiport/40
  ratechange_splitcomp/37 -> splitcomp_multiport/38
  ratechange_splitcomp/35 -> splitcomp_multiport/36
  ratechange_splitcomp/33 -> splitcomp_multiport/34
  ratechange_splitcomp/46 -> splitcomp_multiport/47
  ratechange_splitcomp/44 -> splitcomp_multiport/45
  ratechange_splitcomp/42 -> splitcomp_multiport/43
  ratechange_splitcomp/40 -> splitcomp_multiport/41
  ratechange_splitcomp/47 -> splitcomp_multiport/48
  ratechange_splitcomp/45 -> splitcomp_multiport/46
  ratechange_splitcomp/43 -> splitcomp_multiport/44
  ratechange_splitcomp/41 -> splitcomp_multiport/42
  splitcomp_multiport/1 -> out0/1
  ratechange_splitcomp/48 -> splitcomp_multiport/49

== system gm_Model/DUT_Test/Goertzel/EnabledGoertzel/streaming_partition_streamed2/Serializer_Subnetwork1 ==
  in0 : Inport  OutDataTypeStr=fixdt(1, 18, 13)  PortDimensions=[1 48]  SampleTime=3.125e-07
  in1 : Inport  Port=2  OutDataTypeStr=fixdt(0, 6, 0)  SampleTime=3.125e-07
  ratechange_splitcomp : Demux  Outputs=48
  splitcomp_multiport : MultiPortSwitch  DataPortOrder=Zero-based contiguous  Inputs=48  DiagnosticForDefault=None  zeroidx=on  OutDataTypeStr=fixdt(1, 18, 13)  SampleTime=3.125e-07  SaturateOnIntegerOverflow=off  InputSameDT=off
  out0 : Outport  OutDataTypeStr=fixdt(1, 18, 13)  SampleTime=3.125e-07
  wires:
  in0/1 -> ratechange_splitcomp/1
  in1/1 -> splitcomp_multiport/1
  ratechange_splitcomp/8 -> splitcomp_multiport/9
  ratechange_splitcomp/2 -> splitcomp_multiport/3
  ratechange_splitcomp/4 -> splitcomp_multiport/5
  ratechange_splitcomp/6 -> splitcomp_multiport/7
  ratechange_splitcomp/7 -> splitcomp_multiport/8
  ratechange_splitcomp/1 -> splitcomp_multiport/2
  ratechange_splitcomp/3 -> splitcomp_multiport/4
  ratechange_splitcomp/5 -> splitcomp_multiport/6
  ratechange_splitcomp/15 -> splitcomp_multiport/16
  ratechange_splitcomp/13 -> splitcomp_multiport/14
  ratechange_splitcomp/11 -> splitcomp_multiport/12
  ratechange_splitcomp/9 -> splitcomp_multiport/10
  ratechange_splitcomp/16 -> splitcomp_multiport/17
  ratechange_splitcomp/14 -> splitcomp_multiport/15
  ratechange_splitcomp/12 -> splitcomp_multiport/13
  ratechange_splitcomp/10 -> splitcomp_multiport/11
  ratechange_splitcomp/23 -> splitcomp_multiport/24
  ratechange_splitcomp/21 -> splitcomp_multiport/22
  ratechange_splitcomp/19 -> splitcomp_multiport/20
  ratechange_splitcomp/17 -> splitcomp_multiport/18
  ratechange_splitcomp/24 -> splitcomp_multiport/25
  ratechange_splitcomp/22 -> splitcomp_multiport/23
  ratechange_splitcomp/20 -> splitcomp_multiport/21
  ratechange_splitcomp/18 -> splitcomp_multiport/19
  ratechange_splitcomp/31 -> splitcomp_multiport/32
  ratechange_splitcomp/29 -> splitcomp_multiport/30
  ratechange_splitcomp/27 -> splitcomp_multiport/28
  ratechange_splitcomp/25 -> splitcomp_multiport/26
  ratechange_splitcomp/32 -> splitcomp_multiport/33
  ratechange_splitcomp/30 -> splitcomp_multiport/31
  ratechange_splitcomp/28 -> splitcomp_multiport/29
  ratechange_splitcomp/26 -> splitcomp_multiport/27
  ratechange_splitcomp/40 -> splitcomp_multiport/41
  ratechange_splitcomp/39 -> splitcomp_multiport/40
  ratechange_splitcomp/37 -> splitcomp_multiport/38
  ratechange_splitcomp/35 -> splitcomp_multiport/36
  ratechange_splitcomp/33 -> splitcomp_multiport/34
  ratechange_splitcomp/38 -> splitcomp_multiport/39
  ratechange_splitcomp/36 -> splitcomp_multiport/37
  ratechange_splitcomp/34 -> splitcomp_multiport/35
  ratechange_splitcomp/41 -> splitcomp_multiport/42
  ratechange_splitcomp/44 -> splitcomp_multiport/45
  ratechange_splitcomp/42 -> splitcomp_multiport/43
  ratechange_splitcomp/45 -> splitcomp_multiport/46
  ratechange_splitcomp/43 -> splitcomp_multiport/44
  ratechange_splitcomp/48 -> splitcomp_multiport/49
  ratechange_splitcomp/46 -> splitcomp_multiport/47
  ratechange_splitcomp/47 -> splitcomp_multiport/48
  splitcomp_multiport/1 -> out0/1

== system gm_Model/DUT_Test/Goertzel/EnabledGoertzel/streaming_partition_streamed2/Serializer_Subnetwork2 ==
  in0 : Inport  OutDataTypeStr=fixdt(1, 18, 13)  PortDimensions=[1 48]  SampleTime=3.125e-07
  in1 : Inport  Port=2  OutDataTypeStr=fixdt(0, 6, 0)  SampleTime=3.125e-07
  ratechange_splitcomp : Demux  Outputs=48
  splitcomp_multiport : MultiPortSwitch  DataPortOrder=Zero-based contiguous  Inputs=48  DiagnosticForDefault=None  zeroidx=on  OutDataTypeStr=fixdt(1, 18, 13)  SampleTime=3.125e-07  SaturateOnIntegerOverflow=off  InputSameDT=off
  out0 : Outport  OutDataTypeStr=fixdt(1, 18, 13)  SampleTime=3.125e-07
  wires:
  in1/1 -> splitcomp_multiport/1
  in0/1 -> ratechange_splitcomp/1
  ratechange_splitcomp/2 -> splitcomp_multiport/3
  ratechange_splitcomp/4 -> splitcomp_multiport/5
  ratechange_splitcomp/6 -> splitcomp_multiport/7
  ratechange_splitcomp/1 -> splitcomp_multiport/2
  ratechange_splitcomp/3 -> splitcomp_multiport/4
  ratechange_splitcomp/5 -> splitcomp_multiport/6
  ratechange_splitcomp/13 -> splitcomp_multiport/14
  ratechange_splitcomp/11 -> splitcomp_multiport/12
  ratechange_splitcomp/9 -> splitcomp_multiport/10
  ratechange_splitcomp/7 -> splitcomp_multiport/8
  ratechange_splitcomp/14 -> splitcomp_multiport/15
  ratechange_splitcomp/12 -> splitcomp_multiport/13
  ratechange_splitcomp/10 -> splitcomp_multiport/11
  ratechange_splitcomp/8 -> splitcomp_multiport/9
  ratechange_splitcomp/21 -> splitcomp_multiport/22
  ratechange_splitcomp/19 -> splitcomp_multiport/20
  ratechange_splitcomp/17 -> splitcomp_multiport/18
  ratechange_splitcomp/15 -> splitcomp_multiport/16
  ratechange_splitcomp/22 -> splitcomp_multiport/23
  ratechange_splitcomp/20 -> splitcomp_multiport/21
  ratechange_splitcomp/18 -> splitcomp_multiport/19
  ratechange_splitcomp/16 -> splitcomp_multiport/17
  ratechange_splitcomp/43 -> splitcomp_multiport/44
  ratechange_splitcomp/29 -> splitcomp_multiport/30
  ratechange_splitcomp/27 -> splitcomp_multiport/28
  ratechange_splitcomp/25 -> splitcomp_multiport/26
  ratechange_splitcomp/23 -> splitcomp_multiport/24
  ratechange_splitcomp/42 -> splitcomp_multiport/43
  ratechange_splitcomp/30 -> splitcomp_multiport/31
  ratechange_splitcomp/28 -> splitcomp_multiport/29
  ratechange_splitcomp/26 -> splitcomp_multiport/27
  ratechange_splitcomp/24 -> splitcomp_multiport/25
  ratechange_splitcomp/47 -> splitcomp_multiport/48
  ratechange_splitcomp/45 -> splitcomp_multiport/46
  ratechange_splitcomp/39 -> splitcomp_multiport/40
  ratechange_splitcomp/37 -> splitcomp_multiport/38
  ratechange_splitcomp/35 -> splitcomp_multiport/36
  ratechange_splitcomp/33 -> splitcomp_multiport/34
  ratechange_splitcomp/31 -> splitcomp_multiport/32
  ratechange_splitcomp/48 -> splitcomp_multiport/49
  ratechange_splitcomp/46 -> splitcomp_multiport/47
  ratechange_splitcomp/44 -> splitcomp_multiport/45
  ratechange_splitcomp/38 -> splitcomp_multiport/39
  ratechange_splitcomp/36 -> splitcomp_multiport/37
  ratechange_splitcomp/34 -> splitcomp_multiport/35
  ratechange_splitcomp/32 -> splitcomp_multiport/33
  ratechange_splitcomp/40 -> splitcomp_multiport/41
  ratechange_splitcomp/41 -> splitcomp_multiport/42
  splitcomp_multiport/1 -> out0/1

== system gm_Model/DUT_Test/Goertzel/EnabledGoertzel/streaming_partition_streamed2/Serializer_Subnetwork3 ==
  in0 : Inport  OutDataTypeStr=fixdt(1, 18, 13)  PortDimensions=[1 48]  SampleTime=3.125e-07
  in1 : Inport  Port=2  OutDataTypeStr=fixdt(0, 6, 0)  SampleTime=3.125e-07
  ratechange_splitcomp : Demux  Outputs=48
  splitcomp_multiport : MultiPortSwitch  DataPortOrder=Zero-based contiguous  Inputs=48  DiagnosticForDefault=None  zeroidx=on  OutDataTypeStr=fixdt(1, 18, 13)  SampleTime=3.125e-07  SaturateOnIntegerOverflow=off  InputSameDT=off
  out0 : Outport  OutDataTypeStr=fixdt(1, 18, 13)  SampleTime=3.125e-07
  wires:
  ratechange_splitcomp/47 -> splitcomp_multiport/48
  ratechange_splitcomp/45 -> splitcomp_multiport/46
  ratechange_splitcomp/43 -> splitcomp_multiport/44
  in1/1 -> splitcomp_multiport/1
  ratechange_splitcomp/48 -> splitcomp_multiport/49
  ratechange_splitcomp/46 -> splitcomp_multiport/47
  ratechange_splitcomp/44 -> splitcomp_multiport/45
  ratechange_splitcomp/42 -> splitcomp_multiport/43
  in0/1 -> ratechange_splitcomp/1
  ratechange_splitcomp/2 -> splitcomp_multiport/3
  ratechange_splitcomp/4 -> splitcomp_multiport/5
  ratechange_splitcomp/1 -> splitcomp_multiport/2
  ratechange_splitcomp/3 -> splitcomp_multiport/4
  ratechange_splitcomp/12 -> splitcomp_multiport/13
  ratechange_splitcomp/10 -> splitcomp_multiport/11
  ratechange_splitcomp/8 -> splitcomp_multiport/9
  ratechange_splitcomp/6 -> splitcomp_multiport/7
  ratechange_splitcomp/11 -> splitcomp_multiport/12
  ratechange_splitcomp/9 -> splitcomp_multiport/10
  ratechange_splitcomp/7 -> splitcomp_multiport/8
  ratechange_splitcomp/5 -> splitcomp_multiport/6
  ratechange_splitcomp/19 -> splitcomp_multiport/20
  ratechange_splitcomp/17 -> splitcomp_multiport/18
  ratechange_splitcomp/15 -> splitcomp_multiport/16
  ratechange_splitcomp/13 -> splitcomp_multiport/14
  ratechange_splitcomp/40 -> splitcomp_multiport/41
  ratechange_splitcomp/20 -> splitcomp_multiport/21
  ratechange_splitcomp/18 -> splitcomp_multiport/19
  ratechange_splitcomp/16 -> splitcomp_multiport/17
  ratechange_splitcomp/14 -> splitcomp_multiport/15
  ratechange_splitcomp/27 -> splitcomp_multiport/28
  ratechange_splitcomp/25 -> splitcomp_multiport/26
  ratechange_splitcomp/23 -> splitcomp_multiport/24
  ratechange_splitcomp/21 -> splitcomp_multiport/22
  ratechange_splitcomp/28 -> splitcomp_multiport/29
  ratechange_splitcomp/26 -> splitcomp_multiport/27
  ratechange_splitcomp/24 -> splitcomp_multiport/25
  ratechange_splitcomp/22 -> splitcomp_multiport/23
  ratechange_splitcomp/35 -> splitcomp_multiport/36
  ratechange_splitcomp/33 -> splitcomp_multiport/34
  ratechange_splitcomp/31 -> splitcomp_multiport/32
  ratechange_splitcomp/29 -> splitcomp_multiport/30
  ratechange_splitcomp/36 -> splitcomp_multiport/37
  ratechange_splitcomp/34 -> splitcomp_multiport/35
  ratechange_splitcomp/32 -> splitcomp_multiport/33
  ratechange_splitcomp/30 -> splitcomp_multiport/31
  ratechange_splitcomp/39 -> splitcomp_multiport/40
  ratechange_splitcomp/37 -> splitcomp_multiport/38
  ratechange_splitcomp/38 -> splitcomp_multiport/39
  ratechange_splitcomp/41 -> splitcomp_multiport/42
  splitcomp_multiport/1 -> out0/1

== system gm_Model/DUT_Test/Goertzel/EnabledGoertzel/streaming_partition_streamed2/counter ==
  globalSchedule : EnablePort  OutDataTypeStr=boolean
  ctr_0_47 : hdlsllib/Sources/HDL Counter  CountType=Count limited  CountInit=double(0)  CountStep=double(1)  CountMax=double(47)  CountFromType=Initial value  CountFrom=double(0)  CountResetPort=off  CountLoadPort=off  CountEnbPort=off  CountDirPort=off  CountHitOutputPort=off  CountDataType=Unsigned  CountWordLen=6  CountFracLen=0  CountSampTime=3.125e-07
  out0 : Outport  OutDataTypeStr=fixdt(0, 6, 0)  SampleTime=3.125e-07  InitialOutput=0
  wires:
  ctr_0_47/1 -> out0/1
